simulink model "avlAerodynamics2D_th"  (R2018b)
settings: Solver=FixedStepAuto  StartTime=0.0  StopTime=length(alphas)  RelTol=1e-3
values from neighbouring files (symbols this model uses):
  ailDefl_deg = 0    [avlAerodynamics2D_ts.m]
  elevDefl_deg = 0    [avlAerodynamics2D_ts.m]
  euler = [0;0;0]    [avlAerodynamics2D_ts.m]
  flpDefl_deg = 0    [avlAerodynamics2D_ts.m]
  rudDefl_deg = 0    [avlAerodynamics2D_ts.m]
  vel_cm = [0;0;0]    [avlAerodynamics2D_ts.m]
libraries: avlAerodynamics2D x1
settings Model: Creator=mcobb  LastModifiedBy=Ayaz

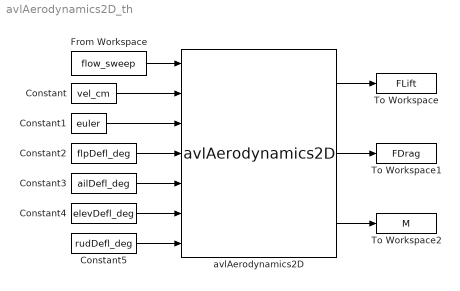
== system avlAerodynamics2D_th ==
  Constant : Constant  Value=vel_cm  VectorParams1D=off
  Constant1 : Constant  Value=euler
  Constant2 : Constant  Value=flpDefl_deg
  Constant3 : Constant  Value=ailDefl_deg
  Constant4 : Constant  Value=elevDefl_deg
  Constant5 : Constant  Value=rudDefl_deg
  From Workspace : FromWorkspace  VariableName=flow_sweep  SampleTime=0
  To Workspace : ToWorkspace  VariableName=FLift  SaveFormat=Timeseries  SampleTime=-1
  To Workspace1 : ToWorkspace  VariableName=FDrag  SaveFormat=Timeseries  SampleTime=-1
  To Workspace2 : ToWorkspace  VariableName=M  SaveFormat=Timeseries  SampleTime=-1
  avlAerodynamics2D : avlAerodynamics2D/avlAerodynamics2D  CLTable=CLtot_2D_Tbl  CDTable=CDtot_2D_Tbl  CMxTable=Cltot_2D_Tbl  CMyTable=Cmtot_2D_Tbl  CMzTable=Cntot_2D_Tbl  CsGainMatrix=k_CS_gain  SRef=Sref  BRef=Bref  CRef=Cref  rho_fluid=rho_fluid
  wires:
  avlAerodynamics2D/3 -> To Workspace2/1
  avlAerodynamics2D/2 -> To Workspace1/1
  avlAerodynamics2D/1 -> To Workspace/1
  Constant4/1 -> avlAerodynamics2D/6
  Constant5/1 -> avlAerodynamics2D/7
  Constant3/1 -> avlAerodynamics2D/5
  Constant2/1 -> avlAerodynamics2D/4
  From Workspace/1 -> avlAerodynamics2D/1
  Constant/1 -> avlAerodynamics2D/2
  Constant1/1 -> avlAerodynamics2D/3
